simulink model "Leader_Acceleration"  (R2022b)
settings: Solver=VariableStepAuto  StartTime=0.0  StopTime=60  RelTol=1e-3
values from neighbouring files (symbols this model uses):
  Ts = 0.1    [MADDPG4_1.m]    (also in MADDPG4__no_rules.m; RL_COMP.m)
  v0_LV = 0.9    [MADDPG4_1.m]    (also in MADDPG4__no_rules.m; RL_COMP.m)
  x0_LV = 3    [MADDPG4_1.m]    (also in MADDPG4__no_rules.m; RL_COMP.m)
libraries: simulink x3
settings Model: Creator=Lenovo  LastModifiedBy=Lenovo
settings DataIOCC: SaveOutput=off  SignalLogging=off  DSMLogging=off  SaveTime=off  ReturnWorkspaceOutputs=off

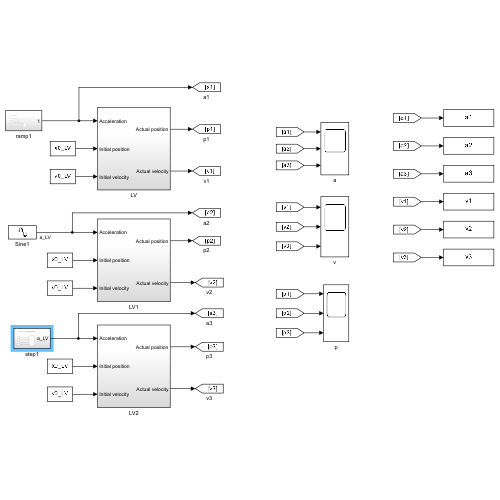
[thumbnail: Simulink's stored preview of the top-level diagram]
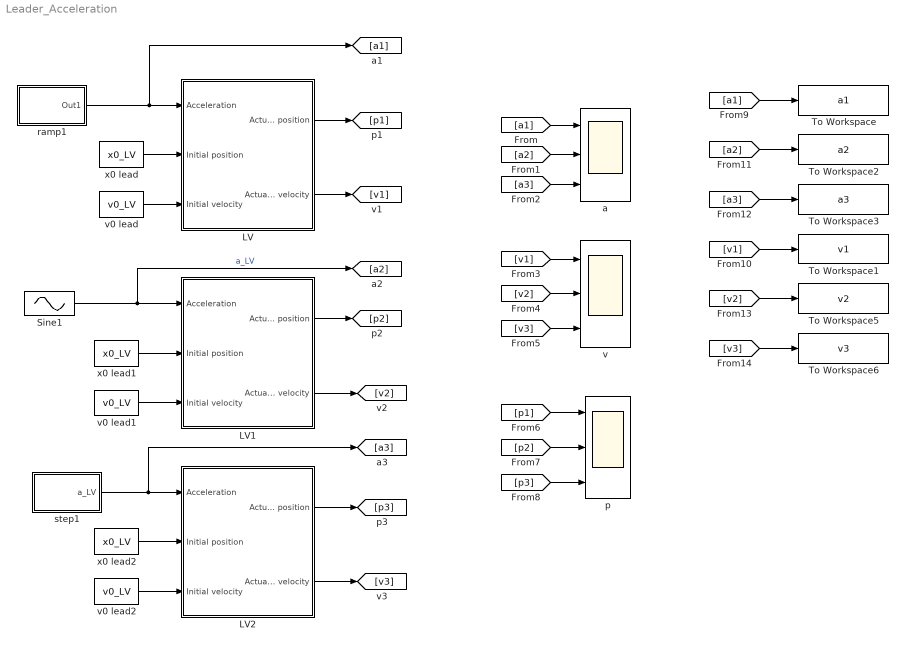
== system Leader_Acceleration ==
  LV : Subsystem
  LV1 : Subsystem
  LV2 : Subsystem
  Sine1 : Sin  Amplitude=0.3  Bias=-0.15  Frequency=2*pi/120  SampleTime=Ts
  To Workspace : ToWorkspace  VariableName=a1  SampleTime=-1
  To Workspace1 : ToWorkspace  VariableName=v1  SampleTime=-1
  To Workspace2 : ToWorkspace  VariableName=a2  SampleTime=-1
  To Workspace3 : ToWorkspace  VariableName=a3  SampleTime=-1
  To Workspace5 : ToWorkspace  VariableName=v2  SampleTime=-1
  To Workspace6 : ToWorkspace  VariableName=v3  SampleTime=-1
  a : Scope  NumInputPorts=3
  p : Scope  NumInputPorts=3
  ramp1 : Subsystem
  step1 : Subsystem
  v : Scope  NumInputPorts=3
  v0 lead : Constant  Value=v0_LV  SampleTime=Ts
  v0 lead1 : Constant  Value=v0_LV  SampleTime=Ts
  v0 lead2 : Constant  Value=v0_LV  SampleTime=Ts
  x0 lead : Constant  Value=x0_LV  SampleTime=Ts
  x0 lead1 : Constant  Value=x0_LV  SampleTime=Ts
  x0 lead2 : Constant  Value=x0_LV  SampleTime=Ts
  wires:
  x0 lead/1 -> LV/2(Initial position)
  v0 lead/1 -> LV/3(Initial velocity)
  ramp1/1(Out1) -> [a1], LV/1(Acceleration)
  x0 lead2/1 -> LV2/2(Initial position)
  v0 lead2/1 -> LV2/3(Initial velocity)
  v0 lead1/1 -> LV1/3(Initial velocity)
  x0 lead1/1 -> LV1/2(Initial position)
  Sine1/1 -> [a2], LV1/1(Acceleration)  "a_LV"
  step1/1(a_LV) -> [a3], LV2/1(Acceleration)
  LV/1(Actual position) -> [p1]
  LV/2(Actual velocity) -> [v1]
  LV2/2(Actual velocity) -> [v3]
  LV1/2(Actual velocity) -> [v2]
  LV1/1(Actual position) -> [p2]
  LV2/1(Actual position) -> [p3]
  [a1] -> To Workspace/1
  [a2] -> To Workspace2/1
  [a3] -> To Workspace3/1
  [v1] -> To Workspace1/1
  [v2] -> To Workspace5/1
  [v3] -> To Workspace6/1
  [v3] -> v/3
  [p3] -> p/3
  [a3] -> a/3
  [a2] -> a/2
  [a1] -> a/1
  [v1] -> v/1
  [v2] -> v/2
  [p2] -> p/2
  [p1] -> p/1

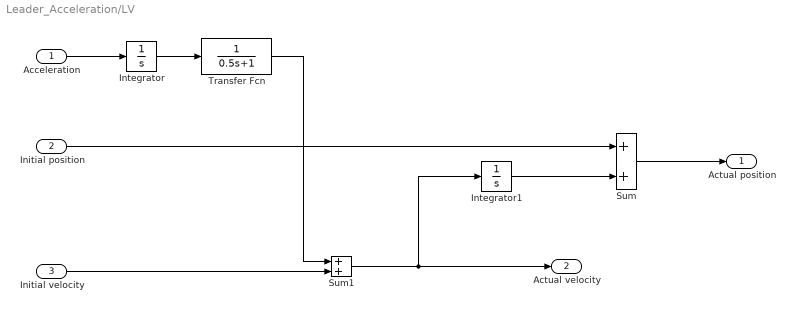
== system Leader_Acceleration/LV ==
  Acceleration : Inport
  Initial position : Inport  Port=2
  Initial velocity : Inport  Port=3
  Integrator : Integrator
  Integrator1 : Integrator
  Sum : Sum
  Sum1 : Sum
  Transfer Fcn : TransferFcn  Denominator=[0.5 1]
  Actual position : Outport  VectorParamsAs1DForOutWhenUnconnected=off
  Actual velocity : Outport  Port=2  VectorParamsAs1DForOutWhenUnconnected=off
  wires:
  Transfer Fcn/1 -> Sum1/1
  Initial velocity/1 -> Sum1/2
  Sum/1 -> Actual position/1
  Integrator/1 -> Transfer Fcn/1
  Sum1/1 -> Integrator1/1, Actual velocity/1
  Acceleration/1 -> Integrator/1
  Initial position/1 -> Sum/1
  Integrator1/1 -> Sum/2

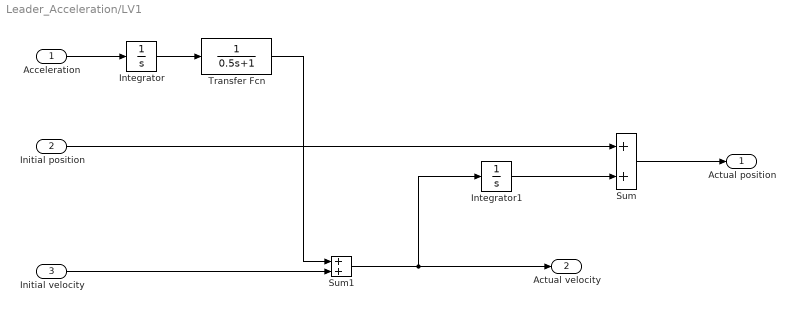
== system Leader_Acceleration/LV1 ==
  Acceleration : Inport
  Initial position : Inport  Port=2
  Initial velocity : Inport  Port=3
  Integrator : Integrator
  Integrator1 : Integrator
  Sum : Sum
  Sum1 : Sum
  Transfer Fcn : TransferFcn  Denominator=[0.5 1]
  Actual position : Outport  VectorParamsAs1DForOutWhenUnconnected=off
  Actual velocity : Outport  Port=2  VectorParamsAs1DForOutWhenUnconnected=off
  wires:
  Integrator1/1 -> Sum/2
  Initial position/1 -> Sum/1
  Acceleration/1 -> Integrator/1
  Sum1/1 -> Actual velocity/1, Integrator1/1
  Integrator/1 -> Transfer Fcn/1
  Sum/1 -> Actual position/1
  Initial velocity/1 -> Sum1/2
  Transfer Fcn/1 -> Sum1/1

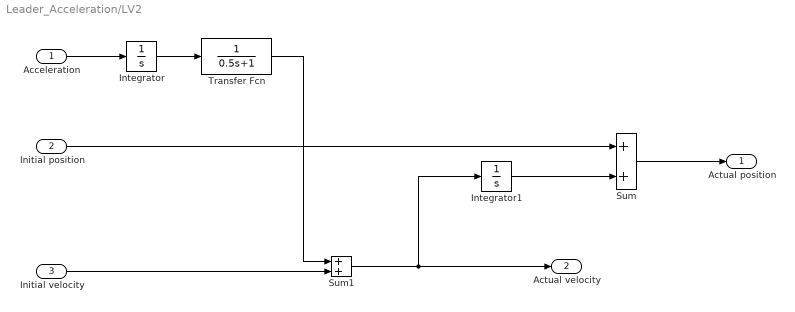
== system Leader_Acceleration/LV2 ==
  Acceleration : Inport
  Initial position : Inport  Port=2
  Initial velocity : Inport  Port=3
  Integrator : Integrator
  Integrator1 : Integrator
  Sum : Sum
  Sum1 : Sum
  Transfer Fcn : TransferFcn  Denominator=[0.5 1]
  Actual position : Outport  VectorParamsAs1DForOutWhenUnconnected=off
  Actual velocity : Outport  Port=2  VectorParamsAs1DForOutWhenUnconnected=off
  wires:
  Transfer Fcn/1 -> Sum1/1
  Initial velocity/1 -> Sum1/2
  Sum/1 -> Actual position/1
  Integrator/1 -> Transfer Fcn/1
  Sum1/1 -> Integrator1/1, Actual velocity/1
  Acceleration/1 -> Integrator/1
  Initial position/1 -> Sum/1
  Integrator1/1 -> Sum/2

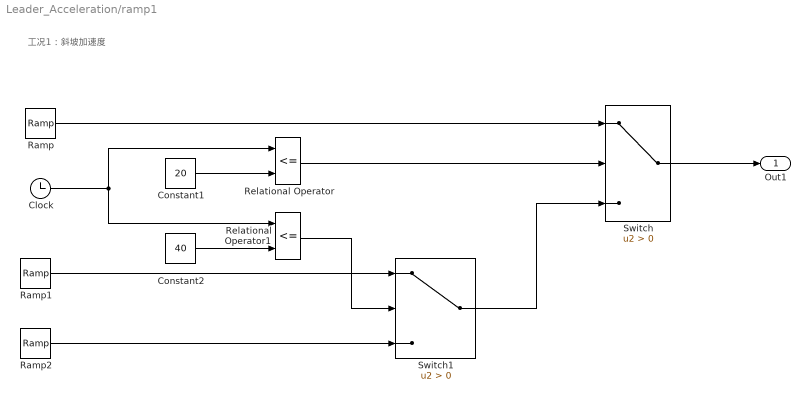
== system Leader_Acceleration/ramp1 ==
  note: 工况1：斜坡加速度
  Clock : Clock
  Constant1 : Constant  Value=20
  Constant2 : Constant  Value=40
  Ramp : simulink/Sources/Ramp  slope=0.01  start=0  InitialOutput=0
  Ramp1 : simulink/Sources/Ramp  slope=-0.01  start=20  InitialOutput=0.2
  Ramp2 : simulink/Sources/Ramp  slope=0  start=40  InitialOutput=0
  Relational Operator : RelationalOperator  Operator=<=  OutDataTypeStr=boolean  RndMeth=Simplest  InputSameDT=off
  Relational Operator1 : RelationalOperator  Operator=<=  OutDataTypeStr=boolean  RndMeth=Simplest  InputSameDT=off
  Switch : Switch  Criteria=u2 > Threshold  SaturateOnIntegerOverflow=off  InputSameDT=off
  Switch1 : Switch  Criteria=u2 > Threshold  SaturateOnIntegerOverflow=off  InputSameDT=off
  Out1 : Outport
  wires:
  Constant1/1 -> Relational Operator/2
  Ramp1/1 -> Switch1/1
  Relational Operator/1 -> Switch/2
  Switch1/1 -> Switch/3
  Relational Operator1/1 -> Switch1/2
  Clock/1 -> Relational Operator1/1, Relational Operator/1
  Ramp/1 -> Switch/1
  Constant2/1 -> Relational Operator1/2
  Ramp2/1 -> Switch1/3
  Switch/1 -> Out1/1

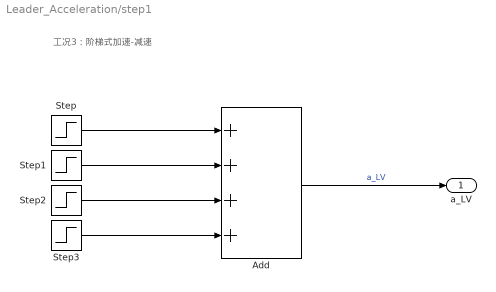
== system Leader_Acceleration/step1 ==
  note: 工况3：阶梯式加速-减速
  Add : Sum  Inputs=++++
  Step : Step  Time=5  SampleTime=0
  Step1 : Step  Time=8  After=-1  SampleTime=0
  Step2 : Step  Time=40  After=-1  SampleTime=0
  Step3 : Step  Time=43  SampleTime=0
  a_LV : Outport
  wires:
  Step2/1 -> Add/3
  Step3/1 -> Add/4
  Step/1 -> Add/1
  Add/1 -> a_LV/1  "a_LV"
  Step1/1 -> Add/2
